simulink model "helloBraccio"  (R2021a)
settings: Solver=FixedStepAuto  StartTime=0.0  StopTime=inf  RelTol=1e-3  EnableMultiTasking=on
libraries: arduinolib x13
settings Model: SILPILModeSetting=veronly  EnablePacing=on  ExtModeTrigDuration=2  Creator=angelo  LastModifiedBy=angelo
settings SolverCC: AutoInsertRateTranBlk=on
settings OptimizationCC: EnhancedBackFolding=on  PassReuseOutputArgsAs=Individual arguments  ZeroExternalMemoryAtStartup=off  ZeroInternalMemoryAtStartup=off  MaxStackSize=64  OptimizeBlockOrder=speed  DifferentSizesBufferReuse=on  OptimizationCustomize=off  EfficientTunableParamExpr=on
settings DebuggingCC: ParameterTunabilityLossMsg=error
settings HardwareCC: ProdBitPerInt=16  ProdBitPerPointer=16  ProdBitPerSizeT=16  ProdBitPerPtrDiffT=16  ProdLargestAtomicFloat=None  ProdWordSize=8  ProdHWDeviceType=Atmel->AVR
settings SFSimCC: MATLABDynamicMemAlloc=off
settings RTWCC: SystemTargetFile=ert.tlc  HardwareBoard=Arduino Mega 2560  TemplateMakefile=ert_default_tmf  Toolchain=Arduino AVR  BuildConfiguration=Faster Runs
settings CodeAppCC: ForceParamTrailComments=on  IgnoreCustomStorageClasses=off  OperatorAnnotations=on  SimulinkDataObjDesc=on  SFDataObjDesc=on  InsertBlockDesc=on
settings ERTTargetCC: SupportContinuousTime=on  SupportVariableSizeSignals=on  ExtModeStaticAllocSize=2048

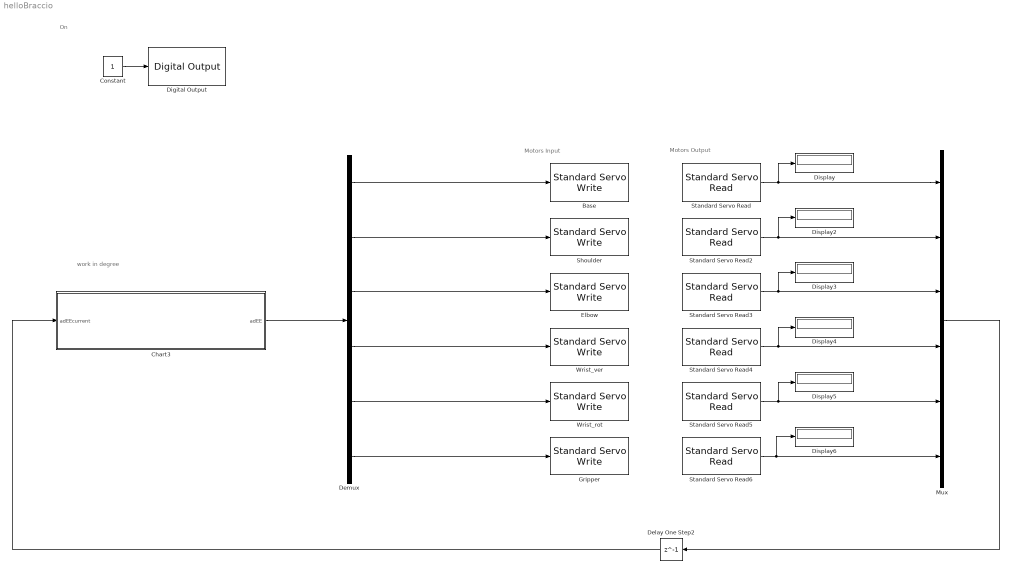
== system helloBraccio ==
  note: On
  note: work in degree
  note: Motors Input
  note: Motors Output
  Base : arduinolib/Standard Servo Write  pinNumber=11  ServoIndex=0  blockPlatform=ARDUINO
  Chart3 : Stateflow chart  TreatAsAtomicUnit=on  SystemSampleTime=0.02
  Constant : Constant
  Delay One Step2 : Delay  DelayLength=1  InitialCondition=[90; 90; 90; 90; 0; 0]
  Demux : Demux  Outputs=6
  Digital Output : arduinolib/Digital Output  pinNumber=12  Direction=output  blockPlatform=arduino
  Display{,2..6} (6 alike) : Display
  Elbow : arduinolib/Standard Servo Write  pinNumber=9  ServoIndex=1  blockPlatform=ARDUINO
  Gripper : arduinolib/Standard Servo Write  pinNumber=3  ServoIndex=2  blockPlatform=ARDUINO
  Mux : Mux  Inputs=6
  Shoulder : arduinolib/Standard Servo Write  pinNumber=10  ServoIndex=3  blockPlatform=ARDUINO
  Standard Servo Read : arduinolib/Standard Servo Read  pinNumber=11  SampleTime=0.02  ServoIndex=0  blockPlatform=ARDUINO
      settings: SourceProductBaseCode=ARDUINO
  Standard Servo Read2 : arduinolib/Standard Servo Read  pinNumber=10  SampleTime=0.02  ServoIndex=3  blockPlatform=ARDUINO
      settings: SourceProductBaseCode=ARDUINO
  Standard Servo Read3 : arduinolib/Standard Servo Read  pinNumber=9  SampleTime=0.02  ServoIndex=1  blockPlatform=ARDUINO
      settings: SourceProductBaseCode=ARDUINO
  Standard Servo Read4 : arduinolib/Standard Servo Read  pinNumber=6  SampleTime=0.02  ServoIndex=4  blockPlatform=ARDUINO
      settings: SourceProductBaseCode=ARDUINO
  Standard Servo Read5 : arduinolib/Standard Servo Read  pinNumber=5  SampleTime=0.02  ServoIndex=5  blockPlatform=ARDUINO
      settings: SourceProductBaseCode=ARDUINO
  Standard Servo Read6 : arduinolib/Standard Servo Read  pinNumber=3  SampleTime=0.02  ServoIndex=2  blockPlatform=ARDUINO
      settings: SourceProductBaseCode=ARDUINO
  Wrist_rot : arduinolib/Standard Servo Write  pinNumber=5  ServoIndex=5  blockPlatform=ARDUINO
  Wrist_ver : arduinolib/Standard Servo Write  pinNumber=6  ServoIndex=4  blockPlatform=ARDUINO
  wires:
  Demux/2 -> Shoulder/1
  Demux/4 -> Wrist_ver/1
  Demux/1 -> Base/1
  Demux/3 -> Elbow/1
  Demux/5 -> Wrist_rot/1
  Constant/1 -> Digital Output/1
  Standard Servo Read5/1 -> Display5/1, Mux/5
  Standard Servo Read3/1 -> Display3/1, Mux/3
  Standard Servo Read/1 -> Display/1, Mux/1
  Standard Servo Read4/1 -> Display4/1, Mux/4
  Standard Servo Read6/1 -> Display6/1, Mux/6
  Standard Servo Read2/1 -> Display2/1, Mux/2
  Demux/6 -> Gripper/1
  Chart3/1(adEE) -> Demux/1
  Delay One Step2/1 -> Chart3/1(adEEcurrent)
  Mux/1 -> Delay One Step2/1

== stateflow chart helloBraccio/Chart3 ==
  settings: executeAtInitialization=1
  state First
    en: adEEdesired = [0; 15; 180; 170; 0; 73];
    during:
    adEE = [
    nextStep(adEEcurrent(1), adEEdesired(1));
    nextStep(adEEcurrent(2), adEEdesired(2));
    nextStep(adEEcurrent(3), adEEdesired(3));
    nextStep(adEEcurrent(4), adEEdesired(4));
    nextStep(adEEcurrent(5), adEEdesired(5));
    nextStep(adEEcurrent(6), adEEdesired(6)); ];
  state Last
    en: adEEdesired = [180; 165; 0; 0; 180; 10];
    during:
    adEE = [
    nextStep(adEEcurrent(1), adEEdesired(1));
    nextStep(adEEcurrent(2), adEEdesired(2));
    nextStep(adEEcurrent(3), adEEdesired(3));
    nextStep(adEEcurrent(4), adEEdesired(4));
    nextStep(adEEcurrent(5), adEEdesired(5));
    nextStep(adEEcurrent(6), adEEdesired(6)); ];
  (default) -> First
  First -> Last : [all(adEEcurrent == adEEdesired)]
  Last -> First : [all(adEEcurrent == adEEdesired)]
  data: current function_input; desired function_input; v function_output; current function_input; desired function_input; v function_output; adEEcurrent input; adEE output; adEEdesired local
  function v = nextStep(current, desired):
    | function v = nextStep(current, desired)
    | if (current < desired)
    |     current = current + 1;
    | end
    | 
    | if (current > desired)
    |     current = current - 1;
    | end
    | 
    | v = current;
    | end
  function v = nextStep(current, desired):
    | function v = nextStep(current, desired)
    | if (current < desired)
    |     current = current + 1;
    | end
    | 
    | if (current > desired)
    |     current = current - 1;
    | end
    | 
    | v = current;
    | end
